simulink model "model"  (R2022b)
settings: Solver=FixedStepDiscrete  StartTime=0.0  StopTime=inf  FixedStep=0.01  RelTol=1e-3
model workspace (MAT data in the model file):
  led1_toggle = Simulink.Parameter
  led1_toggle.Value = 1
  led1_toggle.DataType = 'auto'
  led1_toggle.Complexity = 'real'
  led1_toggle.Dimensions = [1 1]
  led2_toggle = Simulink.Parameter
  led2_toggle.Value = 2
  led2_toggle.DataType = 'auto'
  led2_toggle.Complexity = 'real'
  led2_toggle.Dimensions = [1 1]
  leds_off = Simulink.Parameter
  leds_off.Value = 4
  leds_off.DataType = 'auto'
  leds_off.Complexity = 'real'
  leds_off.Dimensions = [1 1]
  leds_on = Simulink.Parameter
  leds_on.Value = 3
  leds_on.DataType = 'auto'
  leds_on.Complexity = 'real'
  leds_on.Dimensions = [1 1]
settings Model: Creator=Ahmed  LastModifiedBy=Ahmed
settings OptimizationCC: DefaultParameterBehavior=Inlined  UseDivisionForNetSlopeComputation=on  GainParamInheritBuiltInType=on  UseFloatMulNetSlope=on  InlineInvariantSignals=on  PassReuseOutputArgsAs=Individual arguments  ZeroExternalMemoryAtStartup=off  ZeroInternalMemoryAtStartup=off  NoFixptDivByZeroProtection=on  EfficientFloat2IntCast=on  LifeSpan=1  OptimizeBlockOrder=speed  DifferentSizesBufferReuse=on  EfficientTunableParamExpr=on
settings DebuggingCC: ParameterTunabilityLossMsg=error
settings HardwareCC: ProdBitPerPointer=32  ProdBitPerSizeT=32  ProdBitPerPtrDiffT=32  ProdLargestAtomicInteger=Long  ProdLargestAtomicFloat=Double  ProdWordSize=32  ProdLongLongMode=on  ProdHWDeviceType=ARM Compatible->ARM Cortex-M
settings SFSimCC: MATLABDynamicMemAlloc=off
settings RTWCC: Description=Embedded Coder  SystemTargetFile=ert.tlc  TemplateMakefile=ert_default_tmf  GenerateReport=on  Toolchain=LCC-win64 v2.4.1 | gmake (64-bit Windows)  LaunchReport=on
settings CodeAppCC: ForceParamTrailComments=on  IgnoreCustomStorageClasses=off  OperatorAnnotations=on  SimulinkDataObjDesc=on  SFDataObjDesc=on  CustomSymbolStrGlobalVar=rt$N$M  CustomSymbolStrType=$N$M  CustomSymbolStrFcn=$N$M$F  CustomSymbolStrMacro=$N$M  InsertBlockDesc=on
settings ERTTargetCC: TargetLangStandard=C99 (ISO)  GenerateSampleERTMain=on  IncludeMdlTerminateFcn=off  CombineSignalStateStructs=on  SupportAbsoluteTime=off  SupportComplex=off  SupportNonInlinedSFcns=on  InlinedParameterPlacement=NonHierarchical  ERTCustomFileTemplate=example_file_process.tlc  ERTFilePackagingFormat=CompactWithDataFile
settings ConfigComp: DVTestSuiteOptimization=Auto  DVDetectOutOfBounds=on  DVModelReferenceHarness=on  DVHarnessSource=Signal Editor

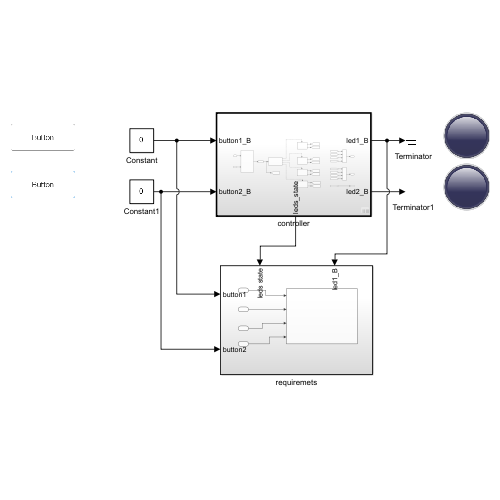
[thumbnail: Simulink's stored preview of the top-level diagram]
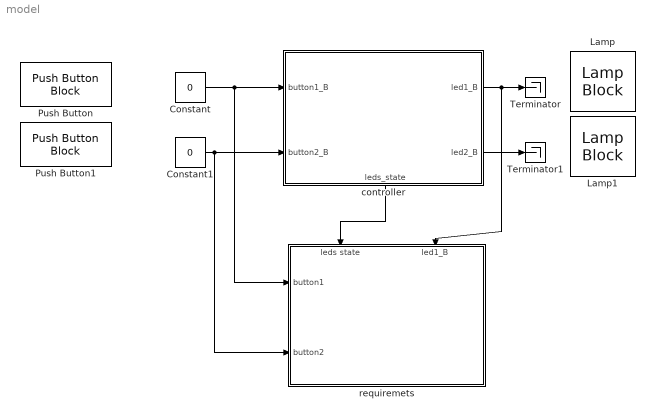
== system model ==
  Constant : Constant  Value=0  OutDataTypeStr=boolean
  Constant1 : Constant  Value=0  OutDataTypeStr=boolean
  Lamp : LampBlock  LabelPosition=Hide
  Lamp1 : LampBlock  LabelPosition=Hide
  Push Button : PushButtonBlock  ButtonType=Latch  OffValue=0.000000
  Push Button1 : PushButtonBlock  ButtonType=Latch  OffValue=0.000000
  Terminator : Terminator
  Terminator1 : Terminator
  controller : Subsystem  TreatAsAtomicUnit=on
      settings: RTWFcnNameOpts=Use subsystem name  PortSchema="{\"entries\":[{\"content\":{\"sides\":[{\"content\":{\"connectorIds\":[\"In1\",\"In2\"]},\"type\":\"ConnectorPlacement.EquallySpacedRectSide\",\"uuid\":\"85f296a8-d7b2-4958-8c3f-8f9af51f5ae9\"},{\"content\":{\"connectorIds\":[\"Out1\",\"Out2\"],\"side\":\"RIGHT\"},\"type\":\"ConnectorPlacement.EquallySpacedRectSide\",\"uuid\":\"f19bd88d-1c2c-44ef-9e20-18e02636a150\"},{\"content\":{\"connectorIds\":[],\"side\":\"TOP\"},\"type\":\"ConnectorPlacement.EquallySpacedRectSide\",\"uuid\":\"d57b5c40-ee15-48c4-8944-b88ec20d146b\"},{\"content\":{\"connectorIds\":[\"Out3\"],\"side\":\"BOTTOM\"},\"type\":\"ConnectorPlacement.EquallySpacedRectSide\",\"uuid\":\"31cc0a18-afd5-4f30-bfb9-5f307c55b616\"}]},\"type\":\"ConnectorPlacement.EquallySpacedConnector\",\"uuid\":\"8a2a85d9-0adc-4706-87df-b71111a90cff\"}],\"packageUris\":[\"http://schema.mathworks.com/mf0/Connector/R2020b\"],\"version\":\"1.0\"}"
  requiremets : Subsystem
      settings: PortSchema="{\"entries\":[{\"content\":{\"sides\":[{\"content\":{\"connectorIds\":[\"In1\",\"In2\"]},\"type\":\"ConnectorPlacement.EquallySpacedRectSide\",\"uuid\":\"7c10ba3e-1223-4a18-a288-42dbb977d165\"},{\"content\":{\"connectorIds\":[],\"side\":\"RIGHT\"},\"type\":\"ConnectorPlacement.EquallySpacedRectSide\",\"uuid\":\"f1a1f911-1aec-4b83-9624-888bf9c4d1f9\"},{\"content\":{\"connectorIds\":[\"In3\",\"In4\"],\"side\":\"TOP\"},\"type\":\"ConnectorPlacement.EquallySpacedRectSide\",\"uuid\":\"2d2579ae-4395-4111-8fda-845b85d924c9\"}]},\"type\":\"ConnectorPlacement.EquallySpacedConnector\",\"uuid\":\"6ece9752-3506-4dc1-8dcb-a64b11d3175b\"}],\"packageUris\":[\"http://schema.mathworks.com/mf0/Connector/R2020b\"],\"version\":\"1.0\"}"
  wires:
  controller/1(led1_B) -> requiremets/4(led1_B), Terminator/1
  controller/2(led2_B) -> Terminator1/1
  Constant/1 -> requiremets/1(button1), controller/1(button1_B)
  Constant1/1 -> controller/2(button2_B), requiremets/2(button2)
  controller/3(leds_state) -> requiremets/3(leds state)

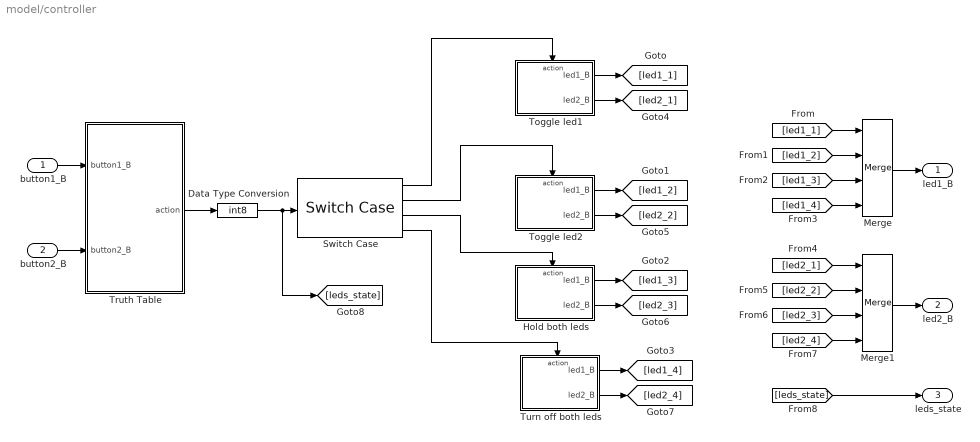
== system model/controller ==
  button1_B : Inport  OutDataTypeStr=boolean
  button2_B : Inport  Port=2  OutDataTypeStr=boolean
  Data Type Conversion : DataTypeConversion  OutDataTypeStr=int8  SaturateOnIntegerOverflow=off  RndMeth=Floor
  Hold both leds : Subsystem  TreatAsAtomicUnit=on
  Merge : Merge  Inputs=4
  Merge1 : Merge  Inputs=4
  Switch Case : SwitchCase  CaseConditions={1,2,3,4}  ShowDefaultCase=off
  Toggle led1 : Subsystem  TreatAsAtomicUnit=on
  Toggle led2 : Subsystem  TreatAsAtomicUnit=on
  Truth Table : Truth Table  TreatAsAtomicUnit=on
  Turn off both leds : Subsystem  TreatAsAtomicUnit=on
  led1_B : Outport  OutDataTypeStr=boolean
  led2_B : Outport  Port=2  OutDataTypeStr=boolean
  leds_state : Outport  Port=3  OutDataTypeStr=int8
  wires:
  Data Type Conversion/1 -> [leds_state], Switch Case/1
  button2_B/1 -> Truth Table/2(button2_B)
  button1_B/1 -> Truth Table/1(button1_B)
  Truth Table/1(action) -> Data Type Conversion/1
  Switch Case/2 -> Toggle led2/Action
  Switch Case/3 -> Hold both leds/Action
  Switch Case/4 -> Turn off both leds/Action
  Toggle led1/1(led1_B) -> [led1_1]
  Toggle led2/1(led1_B) -> [led1_2]
  Hold both leds/1(led1_B) -> [led1_3]
  Turn off both leds/1(led1_B) -> [led1_4]
  Toggle led1/2(led2_B) -> [led2_1]
  Toggle led2/2(led2_B) -> [led2_2]
  Hold both leds/2(led2_B) -> [led2_3]
  Turn off both leds/2(led2_B) -> [led2_4]
  [led1_1] -> Merge/1
  [led1_2] -> Merge/2
  [led1_3] -> Merge/3
  [led1_4] -> Merge/4
  [led2_4] -> Merge1/4
  [led2_3] -> Merge1/3
  [led2_2] -> Merge1/2
  [led2_1] -> Merge1/1
  Merge/1 -> led1_B/1
  Merge1/1 -> led2_B/1
  Switch Case/1 -> Toggle led1/Action
  [leds_state] -> leds_state/1

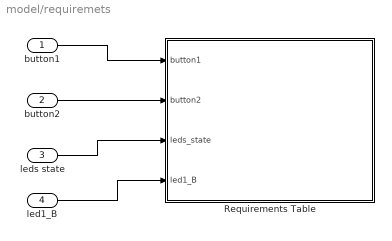
== system model/requiremets ==
  button1 : Inport  OutDataTypeStr=boolean
  button2 : Inport  Port=2  OutDataTypeStr=boolean
  leds state : Inport  Port=3
  led1_B : Inport  Port=4
  Requirements Table : Requirements Table  TreatAsAtomicUnit=on
  wires:
  button1/1 -> Requirements Table/1(button1)
  button2/1 -> Requirements Table/2(button2)
  leds state/1 -> Requirements Table/3(leds_state)
  led1_B/1 -> Requirements Table/4(led1_B)

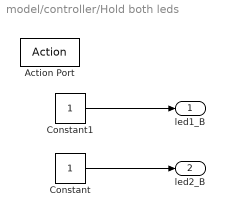
== system model/controller/Hold both leds ==
  Action Port : ActionPort
  Constant : Constant  OutDataTypeStr=boolean
  Constant1 : Constant  OutDataTypeStr=boolean
  led1_B : Outport  OutDataTypeStr=boolean
  led2_B : Outport  Port=2  OutDataTypeStr=boolean
  wires:
  Constant/1 -> led2_B/1
  Constant1/1 -> led1_B/1

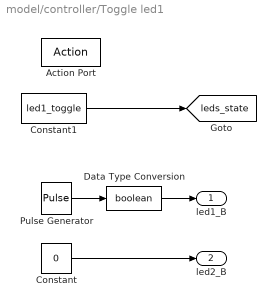
== system model/controller/Toggle led1 ==
  Action Port : ActionPort
  Constant : Constant  Value=0  OutDataTypeStr=boolean
  Constant1 : Constant  Value=led1_toggle  OutDataTypeStr=int8
  Data Type Conversion : DataTypeConversion  OutDataTypeStr=boolean  SaturateOnIntegerOverflow=off  RndMeth=Floor
  Pulse Generator : DiscretePulseGenerator  PulseType=Time based  Period=0.5  PulseWidth=50
  led1_B : Outport  OutDataTypeStr=boolean
  led2_B : Outport  Port=2  OutDataTypeStr=boolean
  tag scope: leds_state=global
  wires:
  Pulse Generator/1 -> Data Type Conversion/1
  Constant/1 -> led2_B/1
  Data Type Conversion/1 -> led1_B/1
  Constant1/1 -> [leds_state]

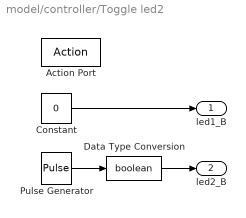
== system model/controller/Toggle led2 ==
  Action Port : ActionPort
  Constant : Constant  Value=0  OutDataTypeStr=boolean
  Data Type Conversion : DataTypeConversion  OutDataTypeStr=boolean  SaturateOnIntegerOverflow=off  RndMeth=Floor
  Pulse Generator : DiscretePulseGenerator  PulseType=Time based  Period=0.5  PulseWidth=50
  led1_B : Outport  OutDataTypeStr=boolean
  led2_B : Outport  Port=2  OutDataTypeStr=boolean
  wires:
  Constant/1 -> led1_B/1
  Pulse Generator/1 -> Data Type Conversion/1
  Data Type Conversion/1 -> led2_B/1

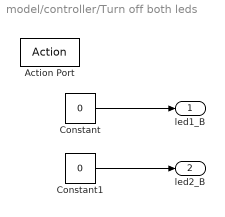
== system model/controller/Turn off both leds ==
  Action Port : ActionPort
  Constant : Constant  Value=0  OutDataTypeStr=boolean
  Constant1 : Constant  Value=0  OutDataTypeStr=boolean
  led1_B : Outport  OutDataTypeStr=boolean
  led2_B : Outport  Port=2  OutDataTypeStr=boolean
  wires:
  Constant/1 -> led1_B/1
  Constant1/1 -> led2_B/1

== matlab function model/controller/Truth Table ==
  data: button1_B input; button2_B input; action output double
function action = fcn(button1_B, button2_B)

aVarTruthTableCondition_1 = false;
aVarTruthTableCondition_2 = false;
aVarTruthTableCondition_3 = false;
aVarTruthTableCondition_4 = false;


% Button1 is pressed

aVarTruthTableCondition_1 = logical(button1_B == true && button2_B == false);

% Button2 is pressed

aVarTruthTableCondition_2 = logical(button2_B == true && button1_B == false);

% Both buttons are pressed

aVarTruthTableCondition_3 = logical(button2_B == true && button1_B == true);

% No pressed buttons

aVarTruthTableCondition_4 = logical(button2_B == false && button1_B == false);

if (aVarTruthTableCondition_1 && ~aVarTruthTableCondition_2 && ~aVarTruthTableCondition_3 && ~aVarTruthTableCondition_4)
    aFcnTruthTableAction_1();
elseif (~aVarTruthTableCondition_1 && aVarTruthTableCondition_2 && ~aVarTruthTableCondition_3 && ~aVarTruthTableCondition_4)
    aFcnTruthTableAction_2();
elseif (~aVarTruthTableCondition_1 && ~aVarTruthTableCondition_2 && aVarTruthTableCondition_3 && ~aVarTruthTableCondition_4)
    aFcnTruthTableAction_3();
elseif (~aVarTruthTableCondition_1 && ~aVarTruthTableCondition_2 && ~aVarTruthTableCondition_3 && aVarTruthTableCondition_4)
    aFcnTruthTableAction_4();
else % Default
    aFcnTruthTableAction_4();
end

function aFcnTruthTableAction_1()

% Toggle led1

action = 1;

function aFcnTruthTableAction_2()

% Toggle led2

action = 2;

function aFcnTruthTableAction_3()

% Hold both led

action = 3;

function aFcnTruthTableAction_4()

% Turn both leds off

action = 4;

== stateflow chart model/requiremets/Requirements Table ==
  (default) -> (junction 1073742325)
  (junction 1073742325) -> (junction 1073742326) : {
      | % SF_REQ_REV_07
      | }
  (junction 1073742326) -> (junction 1073742328) : {
      | % HEADER_ASSIGNMENTS
      |
      | }
  (junction 1073742328) -> (junction 1073742330) : {
      | % START_A_4
      | }
  (junction 1073742330) -> (junction 1073742332) : {
      | }
  (junction 1073742332) -> (junction 1073742334)
  (junction 1073742334) -> (junction 1073742336) : {
      | }
  (junction 1073742336) -> (junction 1073742338) : {
      | % END_A_4
      | }
  (junction 1073742338) -> (junction 1073742340) : {
      | % START_R_1
      | }
  (junction 1073742340) -> (junction 1073742342) : {
      | }
  (junction 1073742342) -> (junction 1073742344)
  (junction 1073742344) -> (junction 1073742346) [order 1] : [((button1 == pressed) && (button2 ~= pressed))]
  (junction 1073742344) -> (junction 1073742352) [order 2]
  (junction 1073742346) -> (junction 1073742348) : {
      | reqtable_postcondition((((leds_state) == (1))) && (((led1_B) == (true))), 'R:1');
      |
      |
      | }
  (junction 1073742348) -> (junction 1073742350) : {
      | }
  (junction 1073742350) -> (junction 1073742352)
  (junction 1073742352) -> (junction 1073742354)
  (junction 1073742354) -> (junction 1073742356) : {
      | % END_R_1
      | }
  (junction 1073742356) -> (junction 1073742358) : {
      | % START_R_7
      | }
  (junction 1073742358) -> (junction 1073742360) : {
      | }
  (junction 1073742360) -> (junction 1073742362)
  (junction 1073742362) -> (junction 1073742364) [order 1] : [((button2 == pressed) && (button1 ~= pressed))]
  (junction 1073742362) -> (junction 1073742370) [order 2]
  (junction 1073742364) -> (junction 1073742366) : {
      | reqtable_postcondition((((leds_state) == (2))) && (((led1_B) == (false))), 'R:2');
      |
      |
      | }
  (junction 1073742366) -> (junction 1073742368) : {
      | }
  (junction 1073742368) -> (junction 1073742370)
  (junction 1073742370) -> (junction 1073742372)
  (junction 1073742372) -> (junction 1073742374) : {
      | % END_R_7
      | }
  (junction 1073742374) -> (junction 1073742376) : {
      | % START_R_10
      | }
  (junction 1073742376) -> (junction 1073742378) : {
      | }
  (junction 1073742378) -> (junction 1073742380)
  (junction 1073742380) -> (junction 1073742382) [order 1] : [((button2 == pressed) && (button1 == pressed))]
  (junction 1073742380) -> (junction 1073742388) [order 2]
  (junction 1073742382) -> (junction 1073742384) : {
      | reqtable_postcondition((((leds_state) == (3))) && (((led1_B) == (true))), 'R:3');
      |
      |
      | }
  (junction 1073742384) -> (junction 1073742386) : {
      | }
  (junction 1073742386) -> (junction 1073742388)
  (junction 1073742388) -> (junction 1073742390)
  (junction 1073742390) -> (junction 1073742392) : {
      | % END_R_10
      | }
  (junction 1073742392) -> (junction 1073742394) : {
      | % START_R_13
      | }
  (junction 1073742394) -> (junction 1073742396) : {
      | }
  (junction 1073742396) -> (junction 1073742398)
  (junction 1073742398) -> (junction 1073742400) [order 1] : [((button2 ~= pressed) && (button1 ~= pressed))]
  (junction 1073742398) -> (junction 1073742406) [order 2]
  (junction 1073742400) -> (junction 1073742402) : {
      | reqtable_postcondition((((leds_state) == (1))) && (((led1_B) == (false))), 'R:4');
      |
      |
      | }
  (junction 1073742402) -> (junction 1073742404) : {
      | }
  (junction 1073742404) -> (junction 1073742406)
  (junction 1073742406) -> (junction 1073742408)
  (junction 1073742408) -> (junction 1073742410) : {
      | % END_R_13
      | }
  data: button1 input boolean; button2 input boolean; leds_state input int8; pressed constant boolean =true; led1_B input boolean
